simulink model "actividad3"  (R2021a)
settings: Solver=ode1  StartTime=0.0  StopTime=500  FixedStep=0.001  RelTol=1e-3
libraries: pid_lib x2
settings Model: Creator=valen  LastModifiedBy=valen

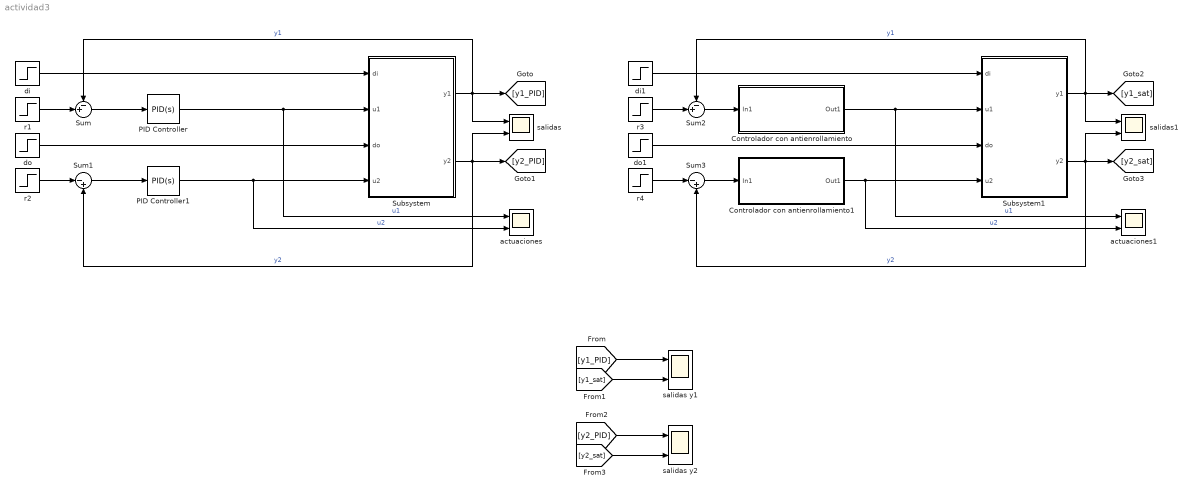
== system actividad3 ==
  Controlador con antienrollamiento : Subsystem  mask{KP=0.8, KI=0.08, tau_p=10}
  Controlador con antienrollamiento1 : Subsystem  mask{KP=0.8, KI=0.08, tau_p=10}
  PID Controller : pid_lib/PID Controller  Controller=PID  Form=Parallel  TimeDomain=Continuous-time  UseExternalTs=off  SampleTime=-1  IntegratorMethod=Forward Euler  FilterMethod=Forward Euler  ControllerParametersSource=internal  P=0.8  I=0.08  D=0  UseFilter=on  N=100  TunerSelectOption=Transfer Function Based (PID Tuner App)  InitialConditionSource=internal  InitialConditionForIntegrator=0  InitialConditionForFilter=0  DifferentiatorICPrevScaledInput=0  ExternalReset=none  TrackingMode=off  Kt=1  LimitOutput=off  SatLimitsSource=internal  UpperSaturationLimit=inf  LowerSaturationLimit=-inf  LinearizeAsGain=on  AntiWindupMode=none  Kb=1  POutMin=[]  POutMax=[]  IOutMin=[]  IOutMax=[]  DOutMin=[]  DOutMax=[]  NOutMin=[]  NOutMax=[]  SumOutMin=[]  SumOutMax=[]  SaturationOutMin=[]  SaturationOutMax=[]  PParamMin=[]  PParamMax=[]  IParamMin=[]  IParamMax=[]  DParamMin=[]  DParamMax=[]  NParamMin=[]  NParamMax=[]  KbParamMin=[]  KbParamMax=[]  KtParamMin=[]  KtParamMax=[]  KbOutMin=[]  KbOutMax=[]  KtOutMin=[]  KtOutMax=[]  IntegratorOutMin=[]  IntegratorOutMax=[]  FilterOutMin=[]  FilterOutMax=[]  SumI1OutMin=[]  SumI1OutMax=[]  SumI2OutMin=[]  SumI2OutMax=[]  SumI3OutMin=[]  SumI3OutMax=[]  SumI4OutMin=[]  SumI4OutMax=[]  SumDOutMin=[]  SumDOutMax=[]  DifferentiatorOutMin=[]  DifferentiatorOutMax=[]  FilterDiffOutCoefMin=[]  FilterDiffOutCoefMax=[]  ReciprocalOutMin=[]  ReciprocalOutMax=[]  SumDenOutMin=[]  SumDenOutMax=[]  SumNumOutMin=[]  SumNumOutMax=[]  DivideOutMin=[]  DivideOutMax=[]  UdiffTsProdOutMin=[]  UdiffTsProdOutMax=[]  NTsProdOutMin=[]  NTsProdOutMax=[]  UintegralTsProdOutMin=[]  UintegralTsProdOutMax=[]  UngainTsProdOutMin=[]  UngainTsProdOutMax=[]  IntegratorContinuousStateAttributes=''  IntegratorStateMustResolveToSignalObject=off  IntegratorRTWStateStorageClass=Auto  FilterContinuousStateAttributes=''  FilterStateMustResolveToSignalObject=off  FilterRTWStateStorageClass=Auto  ParallelPVariant=InternalParameters  IdealPVariant=Disabled  IVariant=InternalParameters  DVariant=InternalParameters  IntegratorVariant=Continuous  SatVariant=Disabled  AWVariant=Passthrough  PCopyVariant=Disabled  TRVariant=Disabled  FdbkBlocksVariant=Forward  IdealPFdbkVariant=Disabled  SatFdbkVariant=Disabled  DerivativeFilterVariant=ContFilter  NVariant=InternalParameters  NCopyVariant=Disabled  FilterICVariant=InternalICsFilter  IntegratorICVariant=InternalICs  ExternalResetVariant=Disabled  TRSumVariant=Passthrough  SumFdbkVariant=Disabled  SumVariant=Sum_PID  TsampFilterVariant=InternalTs  TsampNgainVariant=Passthrough  TsampIntegralVariant=Passthrough  ExternalSaturationOutDataTypeStr=Inherit: Same as second input
  PID Controller1 : pid_lib/PID Controller  Controller=PID  Form=Parallel  TimeDomain=Continuous-time  UseExternalTs=off  SampleTime=-1  IntegratorMethod=Forward Euler  FilterMethod=Forward Euler  ControllerParametersSource=internal  P=0.8  I=0.08  D=0  UseFilter=on  N=100  TunerSelectOption=Transfer Function Based (PID Tuner App)  InitialConditionSource=internal  InitialConditionForIntegrator=0  InitialConditionForFilter=0  DifferentiatorICPrevScaledInput=0  ExternalReset=none  TrackingMode=off  Kt=1  LimitOutput=off  SatLimitsSource=internal  UpperSaturationLimit=inf  LowerSaturationLimit=-inf  LinearizeAsGain=on  AntiWindupMode=none  Kb=1  POutMin=[]  POutMax=[]  IOutMin=[]  IOutMax=[]  DOutMin=[]  DOutMax=[]  NOutMin=[]  NOutMax=[]  SumOutMin=[]  SumOutMax=[]  SaturationOutMin=[]  SaturationOutMax=[]  PParamMin=[]  PParamMax=[]  IParamMin=[]  IParamMax=[]  DParamMin=[]  DParamMax=[]  NParamMin=[]  NParamMax=[]  KbParamMin=[]  KbParamMax=[]  KtParamMin=[]  KtParamMax=[]  KbOutMin=[]  KbOutMax=[]  KtOutMin=[]  KtOutMax=[]  IntegratorOutMin=[]  IntegratorOutMax=[]  FilterOutMin=[]  FilterOutMax=[]  SumI1OutMin=[]  SumI1OutMax=[]  SumI2OutMin=[]  SumI2OutMax=[]  SumI3OutMin=[]  SumI3OutMax=[]  SumI4OutMin=[]  SumI4OutMax=[]  SumDOutMin=[]  SumDOutMax=[]  DifferentiatorOutMin=[]  DifferentiatorOutMax=[]  FilterDiffOutCoefMin=[]  FilterDiffOutCoefMax=[]  ReciprocalOutMin=[]  ReciprocalOutMax=[]  SumDenOutMin=[]  SumDenOutMax=[]  SumNumOutMin=[]  SumNumOutMax=[]  DivideOutMin=[]  DivideOutMax=[]  UdiffTsProdOutMin=[]  UdiffTsProdOutMax=[]  NTsProdOutMin=[]  NTsProdOutMax=[]  UintegralTsProdOutMin=[]  UintegralTsProdOutMax=[]  UngainTsProdOutMin=[]  UngainTsProdOutMax=[]  IntegratorContinuousStateAttributes=''  IntegratorStateMustResolveToSignalObject=off  IntegratorRTWStateStorageClass=Auto  FilterContinuousStateAttributes=''  FilterStateMustResolveToSignalObject=off  FilterRTWStateStorageClass=Auto  ParallelPVariant=InternalParameters  IdealPVariant=Disabled  IVariant=InternalParameters  DVariant=InternalParameters  IntegratorVariant=Continuous  SatVariant=Disabled  AWVariant=Passthrough  PCopyVariant=Disabled  TRVariant=Disabled  FdbkBlocksVariant=Forward  IdealPFdbkVariant=Disabled  SatFdbkVariant=Disabled  DerivativeFilterVariant=ContFilter  NVariant=InternalParameters  NCopyVariant=Disabled  FilterICVariant=InternalICsFilter  IntegratorICVariant=InternalICs  ExternalResetVariant=Disabled  TRSumVariant=Passthrough  SumFdbkVariant=Disabled  SumVariant=Sum_PID  TsampFilterVariant=InternalTs  TsampNgainVariant=Passthrough  TsampIntegralVariant=Passthrough  ExternalSaturationOutDataTypeStr=Inherit: Same as second input
  Subsystem : Subsystem
  Subsystem1 : Subsystem
  Sum : Sum  Inputs=-+|
  Sum1 : Sum  Inputs=|-+
  Sum2 : Sum  Inputs=-+|
  Sum3 : Sum  Inputs=|-+
  actuaciones : Scope  NumInputPorts=2
  actuaciones1 : Scope  NumInputPorts=2
  di : Step  Time=150  After=1.5  SampleTime=0
  di1 : Step  Time=150  After=1.5  SampleTime=0
  do : Step  Time=300  After=2  SampleTime=0
  do1 : Step  Time=300  After=2  SampleTime=0
  r1 : Step  Time=0  After=5  SampleTime=0
  r2 : Step  Time=0  After=3  SampleTime=0
  r3 : Step  Time=0  After=5  SampleTime=0
  r4 : Step  Time=0  After=3  SampleTime=0
  salidas : Scope  NumInputPorts=2
  salidas y1 : Scope  NumInputPorts=2
  salidas y2 : Scope  NumInputPorts=2
  salidas1 : Scope  NumInputPorts=2
  wires:
  PID Controller/1 -> actuaciones/1, Subsystem/2(u1)  "u1"
  PID Controller1/1 -> actuaciones/2, Subsystem/4(u2)  "u2"
  Sum1/1 -> PID Controller1/1
  Subsystem/2(y2) -> [y2_PID], Sum1/2, salidas/2  "y2"
  Subsystem/1(y1) -> [y1_PID], Sum/1, salidas/1  "y1"
  Sum/1 -> PID Controller/1
  di/1 -> Subsystem/1(di)
  do/1 -> Subsystem/3(do)
  r2/1 -> Sum1/1
  r1/1 -> Sum/2
  Sum2/1 -> Controlador con antienrollamiento/1(In1)
  Controlador con antienrollamiento1/1(Out1) -> Subsystem1/4(u2), actuaciones1/2  "u2"
  Subsystem1/2(y2) -> [y2_sat], Sum3/2, salidas1/2  "y2"
  di1/1 -> Subsystem1/1(di)
  Subsystem1/1(y1) -> [y1_sat], Sum2/1, salidas1/1  "y1"
  r4/1 -> Sum3/1
  Controlador con antienrollamiento/1(Out1) -> actuaciones1/1, Subsystem1/2(u1)  "u1"
  r3/1 -> Sum2/2
  Sum3/1 -> Controlador con antienrollamiento1/1(In1)
  do1/1 -> Subsystem1/3(do)
  [y1_PID] -> salidas y1/1
  [y1_sat] -> salidas y1/2
  [y2_sat] -> salidas y2/2
  [y2_PID] -> salidas y2/1

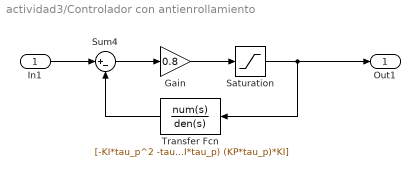
== system actividad3/Controlador con antienrollamiento ==
  In1 : Inport
  Gain : Gain  Gain=0.8
  Saturation : Saturate  UpperLimit=2  LowerLimit=-2
  Sum4 : Sum  Inputs=|+-
  Transfer Fcn : TransferFcn  Numerator=[-KI*tau_p^2 -tau_p*KI]  Denominator=[(KP*tau_p)^2 (KP*tau_p)*(KP+KI*tau_p) (KP*tau_p)*KI]
  Out1 : Outport
  wires:
  In1/1 -> Sum4/1
  Gain/1 -> Saturation/1
  Saturation/1 -> Out1/1, Transfer Fcn/1
  Sum4/1 -> Gain/1
  Transfer Fcn/1 -> Sum4/2

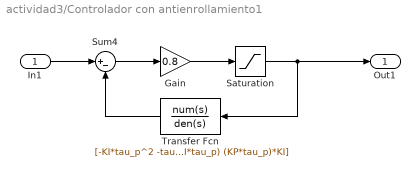
== system actividad3/Controlador con antienrollamiento1 ==
  In1 : Inport
  Gain : Gain  Gain=0.8
  Saturation : Saturate  UpperLimit=2  LowerLimit=-2
  Sum4 : Sum  Inputs=|+-
  Transfer Fcn : TransferFcn  Numerator=[-KI*tau_p^2 -tau_p*KI]  Denominator=[(KP*tau_p)^2 (KP*tau_p)*(KP+KI*tau_p) (KP*tau_p)*KI]
  Out1 : Outport
  wires:
  In1/1 -> Sum4/1
  Gain/1 -> Saturation/1
  Saturation/1 -> Out1/1, Transfer Fcn/1
  Sum4/1 -> Gain/1
  Transfer Fcn/1 -> Sum4/2

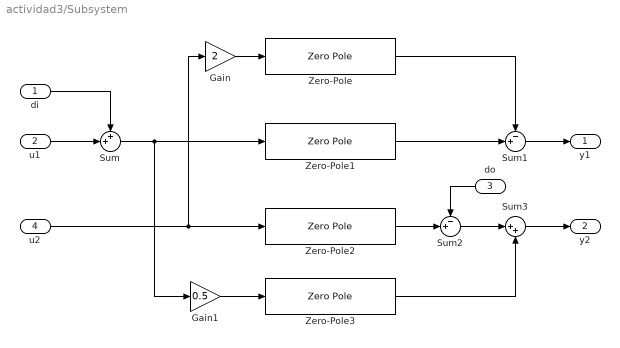
== system actividad3/Subsystem ==
  di : Inport
  u1 : Inport  Port=2
  do : Inport  Port=3
  u2 : Inport  Port=4
  Gain : Gain  Gain=2
  Gain1 : Gain  Gain=0.5
  Sum : Sum  Inputs=++|
  Sum1 : Sum  Inputs=-+|
  Sum2 : Sum  Inputs=-+|
  Sum3 : Sum  Inputs=|++
  Zero-Pole : ZeroPole  Zeros=[0]  Poles=[0 -0.1]  Gain=[0.0125]
  Zero-Pole1 : ZeroPole  Zeros=[-0.05]  Poles=[0 -0.1]  Gain=[0.25]
  Zero-Pole2 : ZeroPole  Zeros=[-0.05]  Poles=[0 -0.1]  Gain=[-0.25]
  Zero-Pole3 : ZeroPole  Zeros=[0]  Poles=[0 -0.1]  Gain=[0.0125]
  y1 : Outport
  y2 : Outport  Port=2
  wires:
  Zero-Pole2/1 -> Sum2/2
  u1/1 -> Sum/2
  di/1 -> Sum/1
  Sum/1 -> Zero-Pole1/1, Gain1/1
  Zero-Pole1/1 -> Sum1/2
  u2/1 -> Gain/1, Zero-Pole2/1
  Sum2/1 -> Sum3/1
  Zero-Pole/1 -> Sum1/1
  Sum3/1 -> y2/1
  Zero-Pole3/1 -> Sum3/2
  do/1 -> Sum2/1
  Gain1/1 -> Zero-Pole3/1
  Gain/1 -> Zero-Pole/1
  Sum1/1 -> y1/1

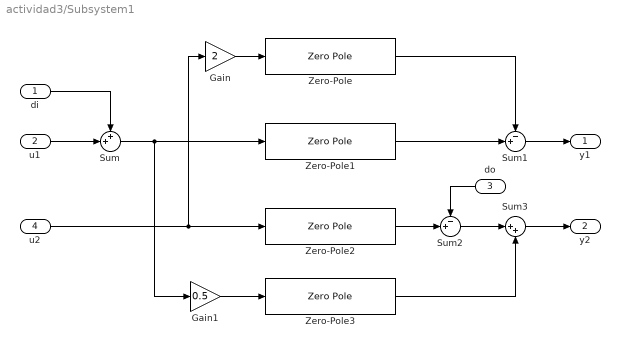
== system actividad3/Subsystem1 ==
  di : Inport
  u1 : Inport  Port=2
  do : Inport  Port=3
  u2 : Inport  Port=4
  Gain : Gain  Gain=2
  Gain1 : Gain  Gain=0.5
  Sum : Sum  Inputs=++|
  Sum1 : Sum  Inputs=-+|
  Sum2 : Sum  Inputs=-+|
  Sum3 : Sum  Inputs=|++
  Zero-Pole : ZeroPole  Zeros=[0]  Poles=[0 -0.1]  Gain=[0.0125]
  Zero-Pole1 : ZeroPole  Zeros=[-0.05]  Poles=[0 -0.1]  Gain=[0.25]
  Zero-Pole2 : ZeroPole  Zeros=[-0.05]  Poles=[0 -0.1]  Gain=[-0.25]
  Zero-Pole3 : ZeroPole  Zeros=[0]  Poles=[0 -0.1]  Gain=[0.0125]
  y1 : Outport
  y2 : Outport  Port=2
  wires:
  Zero-Pole2/1 -> Sum2/2
  u1/1 -> Sum/2
  di/1 -> Sum/1
  Sum/1 -> Zero-Pole1/1, Gain1/1
  Zero-Pole1/1 -> Sum1/2
  u2/1 -> Gain/1, Zero-Pole2/1
  Sum2/1 -> Sum3/1
  Zero-Pole/1 -> Sum1/1
  Sum3/1 -> y2/1
  Zero-Pole3/1 -> Sum3/2
  do/1 -> Sum2/1
  Gain1/1 -> Zero-Pole3/1
  Gain/1 -> Zero-Pole/1
  Sum1/1 -> y1/1
